simulink model "Abbes_conroller"  (R2021b)
settings: Solver=VariableStepAuto  StartTime=0.0  StopTime=10.0  RelTol=1e-3
settings Model: Creator=bober2  LastModifiedBy=bober2
settings SolverCC: ZeroCrossControl=DisableAll  ZeroCrossAlgorithm=Adaptive
settings DebuggingCC: IgnoredZcDiagnostic=none

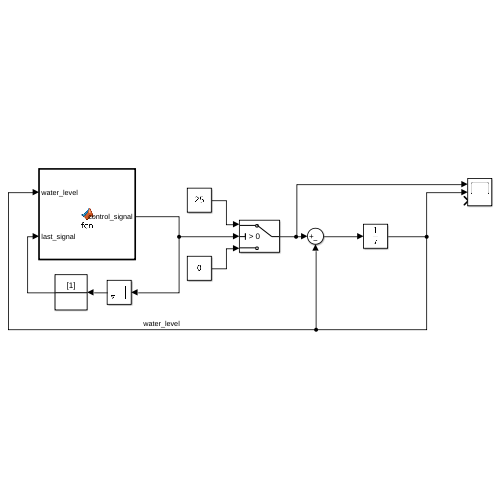
[thumbnail: Simulink's stored preview of the top-level diagram]
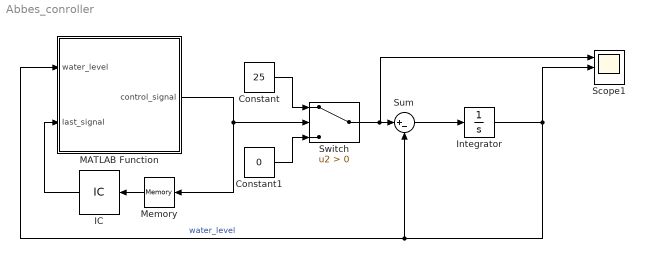
== system Abbes_conroller ==
  Constant : Constant  Value=25
  Constant1 : Constant  Value=0
  IC : InitialCondition
  Integrator : Integrator
  MATLAB Function : MATLAB Function  TreatAsAtomicUnit=on
  Memory : Memory
  Scope1 : Scope  NumInputPorts=3
  Sum : Sum  Inputs=|+-
  Switch : Switch  Criteria=u2 > Threshold
  wires:
  Integrator/1 -> Sum/2, MATLAB Function/1(water_level), Scope1/2  "water_level"
  MATLAB Function/1(control_signal) -> Switch/2, Memory/1
  Memory/1 -> IC/1
  IC/1 -> MATLAB Function/2(last_signal)
  Switch/1 -> Scope1/1, Sum/1
  Constant1/1 -> Switch/3
  Constant/1 -> Switch/1
  Sum/1 -> Integrator/1

== matlab function Abbes_conroller/MATLAB Function ==
  data: control_signal output; water_level input; last_signal input
function control_signal  = fcn(water_level, last_signal)

if water_level < 10
    control_signal = 1;

elseif water_level > 15
    control_signal = 0;

else 
    control_signal = last_signal ;
end 

% 
% if control_signal == 1
%     control = 25;
% else 
%     control = 0 ; 
% end
% 
% flow = (control - water_level);
end
